simulink model "lab7_g2_number2slx"  (R2016a)
settings: Solver=VariableStepAuto  StartTime=0.0  StopTime=10.0  RelTol=1e-3
settings Model: Creator=Student  LastModifiedBy=AIUB

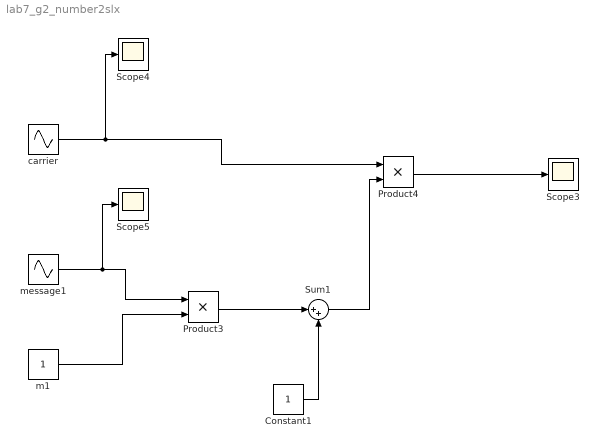
== system lab7_g2_number2slx ==
  " carrier" : Sin  Frequency=2*pi*25  SampleTime=1/5000
  " message1" : Sin  Frequency=2*pi  SampleTime=1/5000
  Constant1 : Constant
  Product3 : Product
  Product4 : Product
  Scope3 : Scope
  Scope4 : Scope
  Scope5 : Scope
  Sum1 : Sum  Inputs=|++
  m1 : Constant
  wires:
  " carrier"/1 -> Scope4/1, Product4/1
  " message1"/1 -> Scope5/1, Product3/1
  m1/1 -> Product3/2
  Product3/1 -> Sum1/1
  Constant1/1 -> Sum1/2
  Sum1/1 -> Product4/2
  Product4/1 -> Scope3/1
